simulink model "position_pid"  (R2025b)
settings: Solver=ode45  StartTime=0.0  StopTime=3  MaxStep=0.005  RelTol=1e-3
InitFcn:
  | addpath(fileparts(get_param(bdroot, 'FileName')))
libraries: slpidlib x1
settings Model: Creator=derekg  LastModifiedBy=derekg

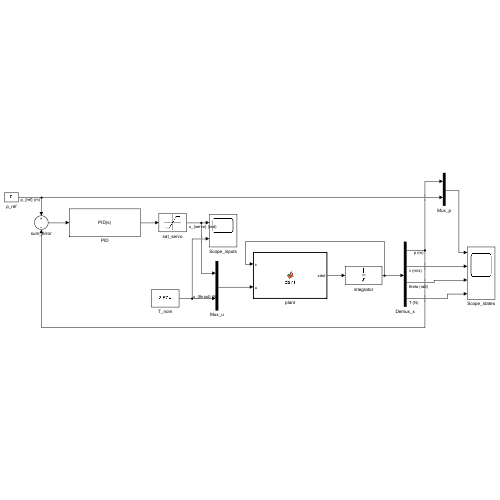
[thumbnail: Simulink's stored preview of the top-level diagram]
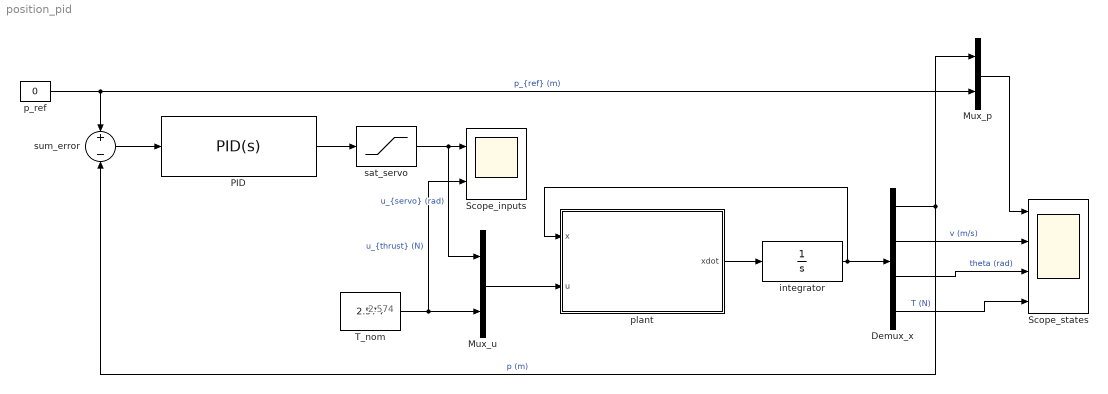
== system position_pid ==
  note: 2.574
  Demux_x : Demux
  Mux_p : Mux  Inputs=2
  Mux_u : Mux  Inputs=2
  PID : slpidlib/PID Controller  Controller=PID  Form=Parallel  TimeDomain=Continuous-time  UseExternalTs=off  SampleTime=-1  IntegratorMethod=Forward Euler  FilterMethod=Forward Euler  ControllerParametersSource=internal  P=3.00161664907217  I=0.263571605759533  UseKiTs=off  D=1.31144510472063  UseExternalDerivativeSource=off  N=1.8234120333855  UseFilter=on  TunerSelectOption=Transfer Function Based (PID Tuner App)  InitialConditionSource=internal  InitialConditionForIntegrator=0  InitialConditionForFilter=0  DifferentiatorICPrevScaledInput=0  ExternalReset=none  TrackingMode=off  Kt=1  LimitOutput=off  SatLimitsSource=internal  UpperSaturationLimit=inf  LowerSaturationLimit=-inf  LinearizeAsGain=on  AntiWindupMode=none  Kb=1  LimitIntegrator=off  UpperIntegratorSaturationLimit=inf  LowerIntegratorSaturationLimit=-inf  POutMin=[]  POutMax=[]  IOutMin=[]  IOutMax=[]  DOutMin=[]  DOutMax=[]  NOutMin=[]  NOutMax=[]  SumOutMin=[]  SumOutMax=[]  SaturationOutMin=[]  SaturationOutMax=[]  PParamMin=[]  PParamMax=[]  IParamMin=[]  IParamMax=[]  DParamMin=[]  DParamMax=[]  NParamMin=[]  NParamMax=[]  KbParamMin=[]  KbParamMax=[]  KtParamMin=[]  KtParamMax=[]  KbOutMin=[]  KbOutMax=[]  KtOutMin=[]  KtOutMax=[]  IntegratorOutMin=[]  IntegratorOutMax=[]  FilterOutMin=[]  FilterOutMax=[]  SumI1OutMin=[]  SumI1OutMax=[]  SumI2OutMin=[]  SumI2OutMax=[]  SumI3OutMin=[]  SumI3OutMax=[]  SumI4OutMin=[]  SumI4OutMax=[]  SumDOutMin=[]  SumDOutMax=[]  DifferentiatorOutMin=[]  DifferentiatorOutMax=[]  FilterDiffOutCoefMin=[]  FilterDiffOutCoefMax=[]  ReciprocalOutMin=[]  ReciprocalOutMax=[]  SumDenOutMin=[]  SumDenOutMax=[]  SumNumOutMin=[]  SumNumOutMax=[]  DivideOutMin=[]  DivideOutMax=[]  UdiffTsProdOutMin=[]  UdiffTsProdOutMax=[]  NTsProdOutMin=[]  NTsProdOutMax=[]  UintegralTsProdOutMin=[]  UintegralTsProdOutMax=[]  UngainTsProdOutMin=[]  UngainTsProdOutMax=[]  ClampingZeroOutDataTypeStr=Inherit: Inherit via back propagation  ClampingZeroOutMin=[]  ClampingZeroOutMax=[]  FilterDenConstantOutDataTypeStr=Inherit: Inherit via back propagation  FilterDenConstantOutMin=[]  FilterDenConstantOutMax=[]  PCopyOutDataTypeStr=Inherit: Inherit via back propagation  PCopyOutMin=[]  PCopyOutMax=[]  NCopyOutDataTypeStr=Inherit: Inherit via back propagation  NCopyOutMin=[]  NCopyOutMax=[]  IntegratorContinuousStateAttributes=''  IntegratorStateMustResolveToSignalObject=off  IntegratorRTWStateStorageClass=Auto  FilterContinuousStateAttributes=''  FilterStateMustResolveToSignalObject=off  FilterRTWStateStorageClass=Auto  ParallelPVariant=InternalParameters  IdealPVariant=Disabled  IVariant=InternalParameters  DVariant=InternalParameters  IntegratorVariant=Continuous  SatVariant=Disabled  AWVariant=Passthrough  PCopyVariant=Disabled  TRVariant=Disabled  FdbkBlocksVariant=Forward  IdealPFdbkVariant=Disabled  SatFdbkVariant=Disabled  DerivativeFilterVariant=ContFilter  NVariant=InternalParameters  NCopyVariant=Disabled  FilterICVariant=InternalICsFilter  IntegratorICVariant=InternalICs  ExternalResetVariant=Disabled  TRSumVariant=Passthrough  SumFdbkVariant=Disabled  SumVariant=Sum_PID  TsampFilterVariant=InternalTs  TsampNgainVariant=Passthrough  TsampIntegralVariant=Disabled_SignalSpec  ExternalSaturationOutDataTypeStr=Inherit: Same as second input  DerivativeSourceVariant=ErrorSignal  PreIntVariant=InternalPreInt
  Scope_inputs : Scope  NumInputPorts=2
      settings: ActiveDisplayYMinimum=-1.9844768416565217  ActiveDisplayYMaximum=3.965690398740529
  Scope_states : Scope  NumInputPorts=4
      settings: ActiveDisplayYMinimum=-0.10754018020061107  ActiveDisplayYMaximum=0.062728174962483646
  T_nom : Constant  Value=2.574
  integrator : Integrator  InitialCondition=[0.15; 0; 0; 2.574]
  p_ref : Constant  Value=0
  plant : MATLAB Function  TreatAsAtomicUnit=on
  sat_servo : Saturate  UpperLimit=pi/3  LowerLimit=-pi/3
  sum_error : Sum  Inputs=+-
  wires:
  integrator/1 -> plant/1(x), Demux_x/1
  Mux_u/1 -> plant/2(u)
  PID/1 -> sat_servo/1
  p_ref/1 -> sum_error/1, Mux_p/2  "p_{ref} (m)"
  sum_error/1 -> PID/1
  sat_servo/1 -> Mux_u/1, Scope_inputs/1  "u_{servo} (rad)"
  T_nom/1 -> Scope_inputs/2, Mux_u/2  "u_{thrust} (N)"
  plant/1(xdot) -> integrator/1
  Demux_x/3 -> Scope_states/3  "theta (rad)"
  Demux_x/1 -> sum_error/2, Mux_p/1  "p (m)"
  Demux_x/2 -> Scope_states/2  "v (m/s)"
  Mux_p/1 -> Scope_states/1
  Demux_x/4 -> Scope_states/4  "T (N)"

== matlab function position_pid/plant ==
  data: x input; u input; xdot output
function xdot = plant(x, u)
% Nonlinear EOM: x = [p; v; theta; T],  u = [theta_cmd_rad; T_cmd_N]
m          = 0.4536;
tau_servo  = 0.0244;
tau_thrust = 0.0781;
mu_c       = 0.8158;
v_sign = tanh(x(2) / 0.05);   % smooth sign: avoids chattering at v≈0 (ε = 5 mm/s)
xdot = [x(2);
        (x(4)*sin(x(3)) - mu_c*v_sign) / m;
        (u(1) - x(3)) / tau_servo;
        (u(2) - x(4)) / tau_thrust];
end
